simulink model "payload_model_2D"  (R2021a)
settings: Solver=FixedStepAuto  StartTime=0.0  StopTime=10.0  RelTol=1e-3
undefined symbols (not defined in the file): c, Cdp, g, k, l, mp, mq, rho
settings Model: Creator=francois  LastModifiedBy=esl
settings SolverCC: AlgebraicLoopSolver=TrustRegion
settings DebuggingCC: SFMachineParentedDataDiag=warning

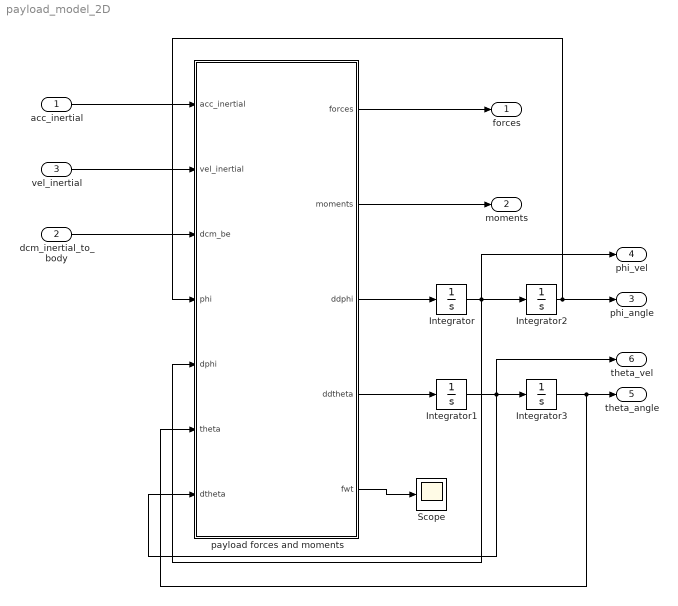
== system payload_model_2D ==
  acc_inertial : Inport  PortDimensions=3
  dcm_inertial_to_body : Inport  Port=2  PortDimensions=[3, 3]
  vel_inertial : Inport  Port=3  PortDimensions=3
  Integrator : Integrator
  Integrator1 : Integrator
  Integrator2 : Integrator  WrapState=on
  Integrator3 : Integrator  WrapState=on
  Scope : Scope
  payload forces and moments : MATLAB Function  TreatAsAtomicUnit=on
  forces : Outport  PortDimensions=3
  moments : Outport  Port=2  PortDimensions=3
  phi_angle : Outport  Port=3  PortDimensions=1
  phi_vel : Outport  Port=4  PortDimensions=1
  theta_angle : Outport  Port=5  PortDimensions=1
  theta_vel : Outport  Port=6  PortDimensions=1
  wires:
  acc_inertial/1 -> payload forces and moments/1(acc_inertial)
  dcm_inertial_to_body/1 -> payload forces and moments/3(dcm_be)
  payload forces and moments/1(forces) -> forces/1
  payload forces and moments/3(ddphi) -> Integrator/1
  Integrator/1 -> payload forces and moments/5(dphi), Integrator2/1, phi_vel/1
  Integrator1/1 -> theta_vel/1, payload forces and moments/7(dtheta), Integrator3/1
  payload forces and moments/4(ddtheta) -> Integrator1/1
  Integrator2/1 -> phi_angle/1, payload forces and moments/4(phi)
  Integrator3/1 -> payload forces and moments/6(theta), theta_angle/1
  payload forces and moments/2(moments) -> moments/1
  vel_inertial/1 -> payload forces and moments/2(vel_inertial)
  payload forces and moments/5(fwt) -> Scope/1

== matlab function payload_model_2D/payload forces and moments ==
  data: acc_inertial input; vel_inertial input; forces output; dcm_be input; phi input; dphi input; theta input; dtheta input; moments output; ddphi output; ddtheta output; mq parameter; mp parameter; l parameter; g parameter; c parameter; k parameter; Cdp parameter; rho parameter; fwt output
function [forces, moments, ddphi, ddtheta, fwt] = payload(acc_inertial, vel_inertial, dcm_be, phi, dphi, theta, dtheta, mq, mp, l, g, c, k, Cdp, rho)

    fwt = 0;
    fwp = 0;
    %% drag forces
    fwt = (0.5*rho*(0 - (vel_inertial(1) + (dtheta*l*cos(phi)*cos(theta) - dphi*l*sin(phi)*sin(theta))))^2*Cdp)*sign(vel_inertial(1));
    fwp = 0.5*rho*(0 - (vel_inertial(2) + dphi*l*cos(phi)))^2*Cdp;
    %fwt = 0;
    %fwp = 0;

    
    %% equations with no damping
    %axi = (mp*cos(phi)*sin(theta)*(l*dphi^2 + l*dtheta^2*cos(phi)^2 + g*cos(theta)*cos(phi)))/(mp + mq);   
    %ayi = (mp*sin(phi)*(l*dphi^2 + l*dtheta^2*cos(phi)^2 + g*cos(theta)*cos(phi)))/(mp + mq);
    %azi = (mp*cos(phi)*cos(theta)*(l*dphi^2 + l*dtheta^2*cos(phi)^2 + g*cos(theta)*cos(phi)))/(mp + mq);
    
    %% equations with c and k
    %axi = (c*dtheta*mp*cos(theta) + c*dtheta*mq*cos(theta) + k*mp*theta*cos(theta) + k*mq*theta*cos(theta) - c*dphi*mp*cos(phi)*sin(phi)*sin(theta) - c*dphi*mq*cos(phi)*sin(phi)*sin(theta) - k*mp*phi*cos(phi)*sin(phi)*sin(theta) - k*mq*phi*cos(phi)*sin(phi)*sin(theta) + dphi^2*l^2*mp*mq*cos(phi)^2*sin(theta) + dtheta^2*l^2*mp*mq*cos(phi)^4*sin(theta) + g*l*mp*mq*cos(phi)^3*cos(theta)*sin(theta))/(l*mq*cos(phi)*(mp + mq));
    %ayi = (c*dphi*mp*cos(phi) + c*dphi*mq*cos(phi) + k*mp*phi*cos(phi) + k*mq*phi*cos(phi) + dphi^2*l^2*mp*mq*sin(phi) + dtheta^2*l^2*mp*mq*cos(phi)^2*sin(phi) + g*l*mp*mq*cos(phi)*cos(theta)*sin(phi))/(l*mq*(mp + mq));
    %azi = -(c*dtheta*mp*sin(theta) + c*dtheta*mq*sin(theta) + k*mp*theta*sin(theta) + k*mq*theta*sin(theta) + c*dphi*mp*cos(phi)*cos(theta)*sin(phi) + c*dphi*mq*cos(phi)*cos(theta)*sin(phi) + k*mp*phi*cos(phi)*cos(theta)*sin(phi) + k*mq*phi*cos(phi)*cos(theta)*sin(phi) - g*l*mp*mq*cos(phi)^3*cos(theta)^2 - dphi^2*l^2*mp*mq*cos(phi)^2*cos(theta) - dtheta^2*l^2*mp*mq*cos(phi)^4*cos(theta))/(l*mq*cos(phi)*(mp + mq));
    
    %% equations with c and k and drag
    axi = (fwt*mp*cos(theta)^2 + fwt*mq*cos(theta)^2 + c*dtheta*mp*cos(theta) + c*dtheta*mq*cos(theta) + k*mp*theta*cos(theta) + k*mq*theta*cos(theta) - fwp*mp*cos(phi)^2*sin(phi)*sin(theta) - fwp*mq*cos(phi)^2*sin(phi)*sin(theta) - c*dphi*mp*cos(phi)*sin(phi)*sin(theta) - c*dphi*mq*cos(phi)*sin(phi)*sin(theta) - k*mp*phi*cos(phi)*sin(phi)*sin(theta) - k*mq*phi*cos(phi)*sin(phi)*sin(theta) + dphi^2*l^2*mp*mq*cos(phi)^2*sin(theta) + dtheta^2*l^2*mp*mq*cos(phi)^4*sin(theta) + g*l*mp*mq*cos(phi)^3*cos(theta)*sin(theta))/(l*mq*cos(phi)*(mp + mq));
    ayi = (fwp*mp*cos(phi)^2 + fwp*mq*cos(phi)^2 + c*dphi*mp*cos(phi) + c*dphi*mq*cos(phi) + k*mp*phi*cos(phi) + k*mq*phi*cos(phi) + dphi^2*l^2*mp*mq*sin(phi) + dtheta^2*l^2*mp*mq*cos(phi)^2*sin(phi) + g*l*mp*mq*cos(phi)*cos(theta)*sin(phi))/(l*mq*(mp + mq));
    azi = -((fwt*mp*sin(2*theta))/2 + (fwt*mq*sin(2*theta))/2 + c*dtheta*mp*sin(theta) + c*dtheta*mq*sin(theta) + k*mp*theta*sin(theta) + k*mq*theta*sin(theta) + fwp*mp*cos(phi)^2*cos(theta)*sin(phi) + fwp*mq*cos(phi)^2*cos(theta)*sin(phi) + c*dphi*mp*cos(phi)*cos(theta)*sin(phi) + c*dphi*mq*cos(phi)*cos(theta)*sin(phi) + k*mp*phi*cos(phi)*cos(theta)*sin(phi) + k*mq*phi*cos(phi)*cos(theta)*sin(phi) - g*l*mp*mq*cos(phi)^3*cos(theta)^2 - dphi^2*l^2*mp*mq*cos(phi)^2*cos(theta) - dtheta^2*l^2*mp*mq*cos(phi)^4*cos(theta))/(l*mq*cos(phi)*(mp + mq));
    %%
    forces = (mq + mp) * dcm_be * [axi; ayi; azi];
    moments = [0; 0; 0];
    
    ddx = acc_inertial(1);
    ddy = acc_inertial(2);
    ddz = acc_inertial(3);
    
    %% equations with no damping
    %ddphi = -(l*cos(phi)*sin(phi)*dtheta^2 + ddy*cos(phi) - ddz*cos(theta)*sin(phi) + g*cos(theta)*sin(phi) - ddx*sin(phi)*sin(theta))/l;
    %ddtheta = -(ddx*cos(theta) - ddz*sin(theta) + g*sin(theta) - 2*dphi*dtheta*l*sin(phi))/(l*cos(phi));
    
    %% equations with c and k
    %ddphi = -(c*dphi + k*phi + ddy*l*mp*cos(phi) + dtheta^2*l^2*mp*cos(phi)*sin(phi) - ddz*l*mp*cos(theta)*sin(phi) + g*l*mp*cos(theta)*sin(phi) - ddx*l*mp*sin(phi)*sin(theta))/(l^2*mp);
    %ddtheta = -(c*dtheta + k*theta + ddx*l*mp*cos(phi)*cos(theta) - ddz*l*mp*cos(phi)*sin(theta) + g*l*mp*cos(phi)*sin(theta) - dphi*dtheta*l^2*mp*sin(2*phi))/(l^2*mp*cos(phi)^2);
    
    %% equations with c and k and drag
    ddphi = -(c*dphi + k*phi + fwp*cos(phi) + ddy*l*mp*cos(phi) + dtheta^2*l^2*mp*cos(phi)*sin(phi) - ddz*l*mp*cos(theta)*sin(phi) + g*l*mp*cos(theta)*sin(phi) - ddx*l*mp*sin(phi)*sin(theta))/(l^2*mp);
    ddtheta = -(c*dtheta + k*theta + fwt*cos(theta) + ddx*l*mp*cos(phi)*cos(theta) - ddz*l*mp*cos(phi)*sin(theta) + g*l*mp*cos(phi)*sin(theta) - dphi*dtheta*l^2*mp*sin(2*phi))/(l^2*mp*cos(phi)^2);

end
